simulink model "TrigSub_lsgBFalling"  (R2018b)
settings: Solver=VariableStepAuto  StartTime=0.0  StopTime=10  FixedStep=0.6  RelTol=1e-3  EnableMultiTasking=on
model workspace (MAT data in the model file):
  AFS = 30
  AS = 0.5
  DT = 5
  cw = 1.3
  g = 9.81
  h0 = 500
  h1 = 150
  m = 85
  rho = 1.2
  v0 = 0
settings Model: Creator=Reichl  LastModifiedBy=Reichl
settings DataIOCC: SaveFormat=Array  TimeSaveName=toutBFalling  OutputSaveName=youtBFalling
settings OptimizationCC: LifeSpan=inf
settings DebuggingCC: SolverPrmCheckMsg=warning  AllowSymbolicDim=off  SFUnexpectedBacktrackingDiag=warning  SFNoUnconditionalDefaultTransitionDiag=warning  SFExecutionAtInitializationDiag=none
settings HardwareCC: ProdBitPerPointer=32  ProdBitPerSizeT=32  ProdBitPerPtrDiffT=32  ProdLargestAtomicFloat=None  ProdIntDivRoundTo=Undefined  ProdEndianess=Unspecified  ProdWordSize=32  ProdHWDeviceType=32-bit Generic
settings ModelReferenceCC: PropagateSignalLabelsOutOfModel=off
settings SFSimCC: SimUseLocalCustomCode=off
settings RTWCC: RTWUseLocalCustomCode=off
settings CodeAppCC: StateflowObjectComments=on
settings GRTTargetCC: TargetLangStandard=C89/C90 (ANSI)  GeneratePreprocessorConditionals=Disable all
settings ConfigComp: CovMetricSettings=dw  CovHtmlReporting=on  CovSaveCumulativeToWorkspaceVar=on  CovSaveSingleToWorkspaceVar=on  CovExternalEMLEnable=off  CovSFcnEnable=off

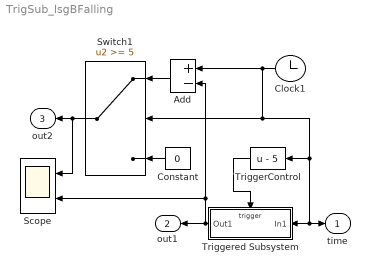
== system TrigSub_lsgBFalling ==
  "     TriggerControl" : Fcn  Expr=u - 5
  Add : Sum  Inputs=+-
  Clock1 : Clock
  Constant : Constant  Value=0
  Scope : Scope  NumInputPorts=2
  Switch1 : Switch  Threshold=5
  Triggered Subsystem : Subsystem  TreatAsAtomicUnit=on
  time : Outport
  out1 : Outport  Port=2
  out2 : Outport  Port=3
  wires:
  "     TriggerControl"/1 -> Triggered Subsystem/Trigger
  Triggered Subsystem/1(Out1) -> Add/2, Scope/2, out1/1
  Switch1/1 -> out2/1, Scope/1
  Clock1/1 -> Switch1/2, time/1, Triggered Subsystem/1(In1), "     TriggerControl"/1, Add/1
  Constant/1 -> Switch1/3
  Add/1 -> Switch1/1

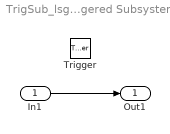
== system TrigSub_lsgBFalling/Triggered Subsystem ==
  In1 : Inport
  Trigger : TriggerPort  TriggerType=falling  VariantControl=Variant
  Out1 : Outport  InitialOutput=-1
  wires:
  In1/1 -> Out1/1
